simulink model "test_YAN_fusion"  (R2020b)
settings: Solver=ode1  StartTime=t0  StopTime=tf  FixedStep=0.004  RelTol=1e-3  EnableMultiTasking=on
values from neighbouring files (symbols this model uses):
  IMU = IN_SENSOR.IMU1    [run_simulation.m]
undefined symbols (not defined in the file or in its folder): accel_x, accel_y, accel_z, airspeed, airspeed1, airspeed2, airspeed3, airspeed_calibrate, airspeed_indicate, airspeed_true, alt_baro, baro1, baro2, BESTPOS, delta_height, delta_lat, delta_lon, dynamic_pressure, EAS2TAS_Algo, flag, Flag, glv, gyro_x, gyro_y, gyro_z, hAcc, headAcc, height, IMU1, IMU1_Control, IMU2, IMU3, IMU4, laserDown1, laserDown2, Lat, Lon, mag1, mag2, mag_x, mag_y, mag_z, nChange, numSv, pDop, radar1, radarLongDown1, radarLongForward1, range, Range, sAcc, SNR, static_pressure, status, strength, temperature, time, ublox1, um482, vAcc ... (+3)
(part 1 of 3)
settings Model: PauseTimes=[10 20]  Creator=sl  LastModifiedBy=sl
settings SolverCC: AutoInsertRateTranBlk=on
settings OptimizationCC: DefaultParameterBehavior=Inlined  EnhancedBackFolding=on  PassReuseOutputArgsAs=Individual arguments  ZeroExternalMemoryAtStartup=off  ZeroInternalMemoryAtStartup=off  MaxStackSize=64  OptimizeBlockOrder=speed  DifferentSizesBufferReuse=on  OptimizationCustomize=off  EfficientTunableParamExpr=on
settings DebuggingCC: MultiTaskCondExecSysMsg=none  ParameterTunabilityLossMsg=error  UnconnectedInputMsg=none  UnconnectedOutputMsg=none  UnconnectedLineMsg=none
settings HardwareCC: ProdBitPerPointer=32  ProdBitPerSizeT=32  ProdBitPerPtrDiffT=32  ProdLargestAtomicInteger=Long  ProdLargestAtomicFloat=Double  ProdWordSize=32  ProdHWDeviceType=ARM Compatible->ARM Cortex
settings SFSimCC: MATLABDynamicMemAlloc=off
settings RTWCC: Description=Embedded Coder  SystemTargetFile=ert.tlc  TemplateMakefile=ert_default_tmf  GenerateReport=on  IncludeHyperlinkInReport=on  LaunchReport=on  GenerateTraceInfo=on  GenerateTraceReport=on  GenerateTraceReportSl=on  GenerateTraceReportSf=on  GenerateTraceReportEml=on
settings CodeAppCC: ForceParamTrailComments=on  IgnoreCustomStorageClasses=off  OperatorAnnotations=on  SimulinkDataObjDesc=on  SFDataObjDesc=on  InsertBlockDesc=on
settings ERTTargetCC: InlinedParameterPlacement=NonHierarchical  ERTCustomFileTemplate=example_file_process.tlc

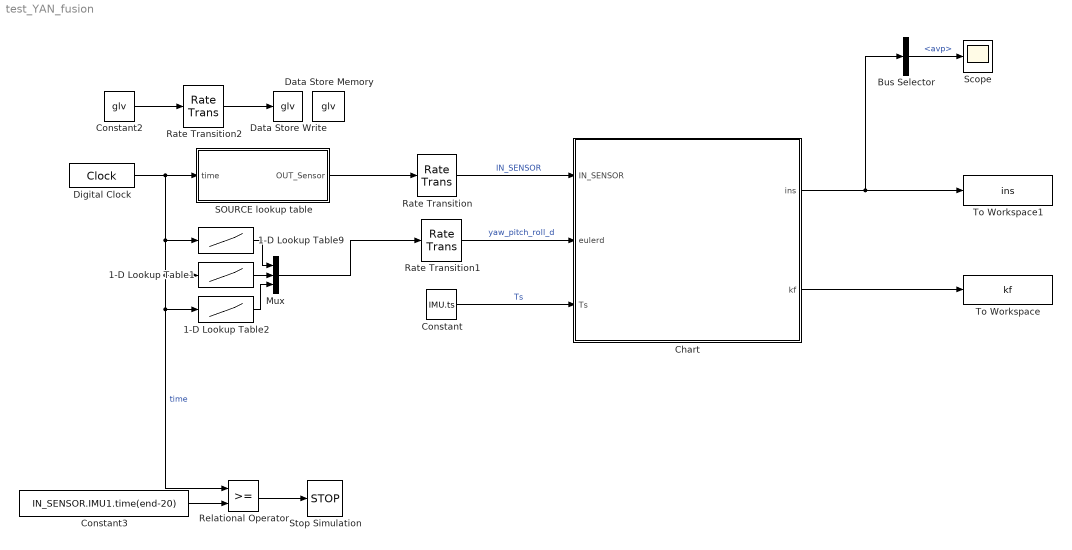
== system test_YAN_fusion ==
  1-D Lookup Table1 : Lookup_n-D  NumberOfTableDimensions=1  BreakpointsForDimension1=FlightLog_Original.Filter.time_cal(1:end-20)  Table=FlightLog_Original.Filter.algo_NAV_pitchd(1:end-20)  InterpMethod=Flat  ExtrapMethod=Clip  InternalRulePriority=Speed  RndMeth=Simplest  InputSameDT=on
  1-D Lookup Table2 : Lookup_n-D  NumberOfTableDimensions=1  BreakpointsForDimension1=FlightLog_Original.Filter.time_cal(1:end-20)  Table=FlightLog_Original.Filter.algo_NAV_rolld(1:end-20)  InterpMethod=Flat  ExtrapMethod=Clip  InternalRulePriority=Speed  RndMeth=Simplest  InputSameDT=on
  1-D Lookup Table9 : Lookup_n-D  NumberOfTableDimensions=1  BreakpointsForDimension1=FlightLog_Original.Filter.time_cal(1:end-20)  Table=FlightLog_Original.Filter.algo_NAV_yawd(1:end-20)  InterpMethod=Flat  ExtrapMethod=Clip  InternalRulePriority=Speed  RndMeth=Simplest  InputSameDT=on
  Bus Selector : BusSelector  OutputSignals=avp
  Chart : Stateflow chart  TreatAsAtomicUnit=on
  Constant : Constant  Value=IMU.ts
  Constant2 : Constant  Value=glv  OutDataTypeStr=Bus: BUS_NAVI_YAN_Glv
  Constant3 : Constant  Value=IN_SENSOR.IMU1.time(end-20)
  Data Store Memory : DataStoreMemory  DataStoreName=glv  ReadBeforeWriteMsg=warning  WriteAfterWriteMsg=warning  WriteAfterReadMsg=warning  ShowAdditionalParam=off  OutDataTypeStr=Bus: BUS_NAVI_YAN_Glv
  Data Store Write : DataStoreWrite  DataStoreName=glv
  Digital Clock : DigitalClock  SampleTime=0.004
  Mux : Mux  Inputs=3
  Rate Transition : RateTransition  OutPortSampleTime=IMU.ts
  Rate Transition1 : RateTransition  OutPortSampleTime=IMU.ts
  Rate Transition2 : RateTransition  OutPortSampleTime=IMU.ts
  Relational Operator : RelationalOperator  OutDataTypeStr=boolean  RndMeth=Simplest
  SOURCE lookup table : Subsystem
  Scope : Scope
  Stop Simulation : Stop
  To Workspace : ToWorkspace  VariableName=kf  SaveFormat=Timeseries  SampleTime=-1
  To Workspace1 : ToWorkspace  VariableName=ins  SaveFormat=Timeseries  SampleTime=-1
  wires:
  Digital Clock/1 -> 1-D Lookup Table1/1, 1-D Lookup Table2/1, Relational Operator/1, 1-D Lookup Table9/1, SOURCE lookup table/1(time)  "time"
  SOURCE lookup table/1(OUT_Sensor) -> Rate Transition/1
  Rate Transition/1 -> Chart/1(IN_SENSOR)  "IN_SENSOR"
  1-D Lookup Table9/1 -> Mux/1
  Constant2/1 -> Rate Transition2/1
  Rate Transition1/1 -> Chart/2(eulerd)  "yaw_pitch_roll_d"
  Rate Transition2/1 -> Data Store Write/1
  Constant/1 -> Chart/3(Ts)  "Ts"
  Chart/2(kf) -> To Workspace/1
  Constant3/1 -> Relational Operator/2
  Relational Operator/1 -> Stop Simulation/1
  Chart/1(ins) -> Bus Selector/1, To Workspace1/1
  Bus Selector/1 -> Scope/1  "<avp>"
  1-D Lookup Table1/1 -> Mux/2
  1-D Lookup Table2/1 -> Mux/3
  Mux/1 -> Rate Transition1/1

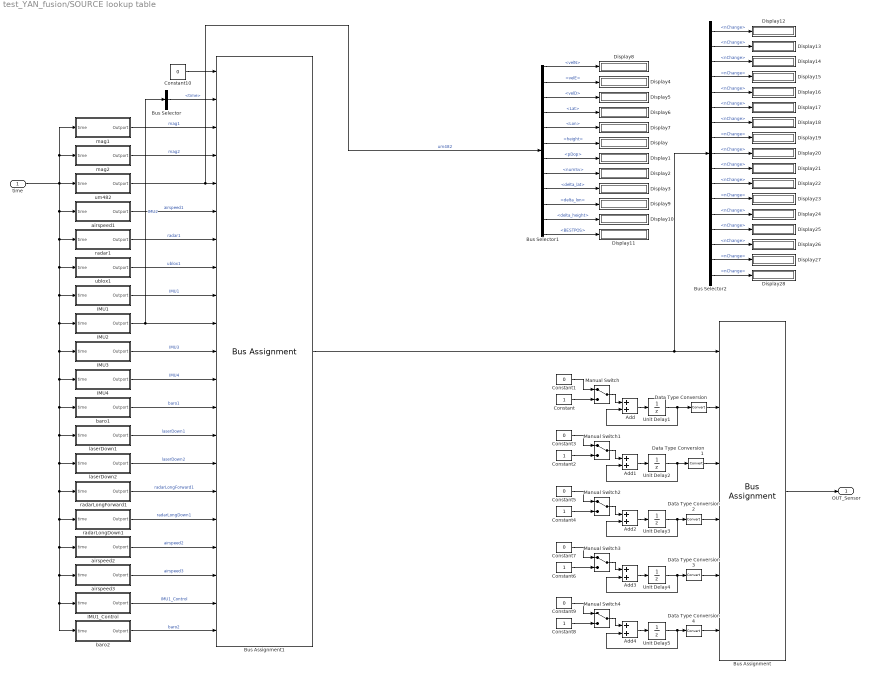
== system test_YAN_fusion/SOURCE lookup table ==
  time : Inport
  Add{,1..4} (5 alike) : Sum
  Bus Assignment : BusAssignment  AssignedSignals=IMU1.nChange,IMU2.nChange,IMU3.nChange,mag1.nChange,mag2.nChange
  Bus Assignment1 : BusAssignment  AssignedSignals=time,mag1,mag2,um482,airspeed1,radar1,ublox1,IMU1,IMU2,IMU3,IMU4,baro1,laserDown1,laserDown2,radarLongForward1,radarLongDown1,airspeed2,airspeed3,IMU1_Control,baro2
  Bus Selector : BusSelector  OutputSignals=time
  Bus Selector1 : BusSelector  OutputSignals=velN,velE,velD,Lat,Lon,height,pDop,numSv,delta_lat,delta_lon,delta_height,BESTPOS
  Bus Selector2 : BusSelector  OutputSignals=mag1.nChange,mag2.nChange,ublox1.nChange,um482.nChange,airspeed1.nChange,airspeed2.nChange,airspeed3.nChange,radar1.nChange,IMU1.nChange,IMU2.nChange,IMU3.nChange,IMU1_Control.nChange,baro1.nChange,laserDown1.nChange,laserDown2.nChange,radarLongForward1.nChange,radarLongDown1.nChange
  Constant{,2,4,6,8} (5 alike) : Constant
  Constant{1,3,5,7,9} (5 alike) : Constant  Value=0
  Constant10 : Constant  Value=0  OutDataTypeStr=Bus: BUS_SENSOR
  Data Type Conversion{,1..4} (5 alike) : DataTypeConversion
  Display{,1..28} (29 alike) : Display
  IMU1 : Subsystem
  IMU1_Control : Subsystem
  IMU2 : Subsystem
  IMU3 : Subsystem
  IMU4 : Subsystem
  Manual Switch{,1..4} (5 alike) : ManualSwitch
  Unit Delay{1..5} (5 alike) : UnitDelay  SampleTime=-1  HasFrameUpgradeWarning=on
  airspeed1 : Subsystem
  airspeed2 : Subsystem
  airspeed3 : Subsystem
  baro1 : Subsystem
  baro2 : Subsystem
  laserDown1 : Subsystem
  laserDown2 : Subsystem
  mag1 : Subsystem
  mag2 : Subsystem
  radar1 : Subsystem
  radarLongDown1 : Subsystem
  radarLongForward1 : Subsystem
  ublox1 : Subsystem
  um482 : Subsystem
  OUT_Sensor : Outport
  wires:
  time/1 -> radarLongForward1/1(time), radarLongDown1/1(time), baro2/1(time), IMU1_Control/1(time), airspeed3/1(time), airspeed2/1(time), laserDown2/1(time), laserDown1/1(time), baro1/1(time), IMU4/1(time), IMU3/1(time), IMU2/1(time), IMU1/1(time), ublox1/1(time), radar1/1(time), airspeed1/1(time), mag2/1(time), mag1/1(time), um482/1(time)
  Bus Selector/1 -> Bus Assignment1/2  "<time>"
  IMU2/1(Outport) -> Bus Assignment1/10, Bus Selector/1  "IMU2"
  ublox1/1(Outport) -> Bus Assignment1/8  "ublox1"
  laserDown2/1(Outport) -> Bus Assignment1/15  "laserDown2"
  IMU3/1(Outport) -> Bus Assignment1/11  "IMU3"
  airspeed2/1(Outport) -> Bus Assignment1/18  "airspeed2"
  um482/1(Outport) -> Bus Assignment1/5, Bus Selector1/1  "um482"
  radarLongDown1/1(Outport) -> Bus Assignment1/17  "radarLongDown1"
  airspeed1/1(Outport) -> Bus Assignment1/6  "airspeed1"
  mag2/1(Outport) -> Bus Assignment1/4  "mag2"
  IMU1/1(Outport) -> Bus Assignment1/9  "IMU1"
  mag1/1(Outport) -> Bus Assignment1/3  "mag1"
  baro1/1(Outport) -> Bus Assignment1/13  "baro1"
  radar1/1(Outport) -> Bus Assignment1/7  "radar1"
  laserDown1/1(Outport) -> Bus Assignment1/14  "laserDown1"
  airspeed3/1(Outport) -> Bus Assignment1/19  "airspeed3"
  IMU1_Control/1(Outport) -> Bus Assignment1/20  "IMU1_Control"
  radarLongForward1/1(Outport) -> Bus Assignment1/16  "radarLongForward1"
  Bus Assignment1/1 -> Bus Selector2/1, Bus Assignment/1
  Bus Selector1/5 -> Display7/1  "<Lon>"
  Bus Selector1/6 -> Display/1  "<height>"
  Bus Selector1/7 -> Display1/1  "<pDop>"
  Bus Selector1/8 -> Display2/1  "<numSv>"
  Bus Selector1/1 -> Display8/1  "<velN>"
  Bus Selector1/2 -> Display4/1  "<velE>"
  Bus Selector1/3 -> Display5/1  "<velD>"
  Bus Selector1/4 -> Display6/1  "<Lat>"
  Bus Selector1/9 -> Display3/1  "<delta_lat>"
  Bus Selector1/10 -> Display9/1  "<delta_lon>"
  Bus Selector1/11 -> Display10/1  "<delta_height>"
  Bus Selector1/12 -> Display11/1  "<BESTPOS>"
  Bus Selector2/1 -> Display12/1  "<nChange>"
  Bus Selector2/2 -> Display13/1  "<nChange>"
  Bus Selector2/3 -> Display14/1  "<nChange>"
  Bus Selector2/4 -> Display15/1  "<nChange>"
  Bus Selector2/5 -> Display16/1  "<nChange>"
  Bus Selector2/6 -> Display17/1  "<nChange>"
  Bus Selector2/7 -> Display18/1  "<nChange>"
  Bus Selector2/8 -> Display19/1  "<nChange>"
  Bus Selector2/9 -> Display20/1  "<nChange>"
  Bus Selector2/10 -> Display21/1  "<nChange>"
  Bus Selector2/11 -> Display22/1  "<nChange>"
  Bus Selector2/12 -> Display23/1  "<nChange>"
  Bus Selector2/13 -> Display24/1  "<nChange>"
  Bus Selector2/14 -> Display25/1  "<nChange>"
  Bus Selector2/15 -> Display26/1  "<nChange>"
  Bus Selector2/16 -> Display27/1  "<nChange>"
  Bus Selector2/17 -> Display28/1  "<nChange>"
  Bus Assignment/1 -> OUT_Sensor/1
  Constant/1 -> Manual Switch/2
  Add/1 -> Unit Delay1/1
  Unit Delay1/1 -> Add/2, Data Type Conversion/1
  Constant1/1 -> Manual Switch/1
  Manual Switch/1 -> Add/1
  Manual Switch1/1 -> Add1/1
  Constant3/1 -> Manual Switch1/1
  Unit Delay2/1 -> Data Type Conversion1/1, Add1/2
  Add1/1 -> Unit Delay2/1
  Constant2/1 -> Manual Switch1/2
  Constant4/1 -> Manual Switch2/2
  Add2/1 -> Unit Delay3/1
  Unit Delay3/1 -> Data Type Conversion2/1, Add2/2
  Constant5/1 -> Manual Switch2/1
  Manual Switch2/1 -> Add2/1
  Data Type Conversion/1 -> Bus Assignment/2
  Data Type Conversion1/1 -> Bus Assignment/3
  Data Type Conversion2/1 -> Bus Assignment/4
  Data Type Conversion3/1 -> Bus Assignment/5
  Manual Switch3/1 -> Add3/1
  Constant7/1 -> Manual Switch3/1
  Unit Delay4/1 -> Add3/2, Data Type Conversion3/1
  Add3/1 -> Unit Delay4/1
  Constant6/1 -> Manual Switch3/2
  Constant8/1 -> Manual Switch4/2
  Add4/1 -> Unit Delay5/1
  Unit Delay5/1 -> Data Type Conversion4/1, Add4/2
  Constant9/1 -> Manual Switch4/1
  Manual Switch4/1 -> Add4/1
  Data Type Conversion4/1 -> Bus Assignment/6
  IMU4/1(Outport) -> Bus Assignment1/12  "IMU4"
  baro2/1(Outport) -> Bus Assignment1/21  "baro2"
  Constant10/1 -> Bus Assignment1/1

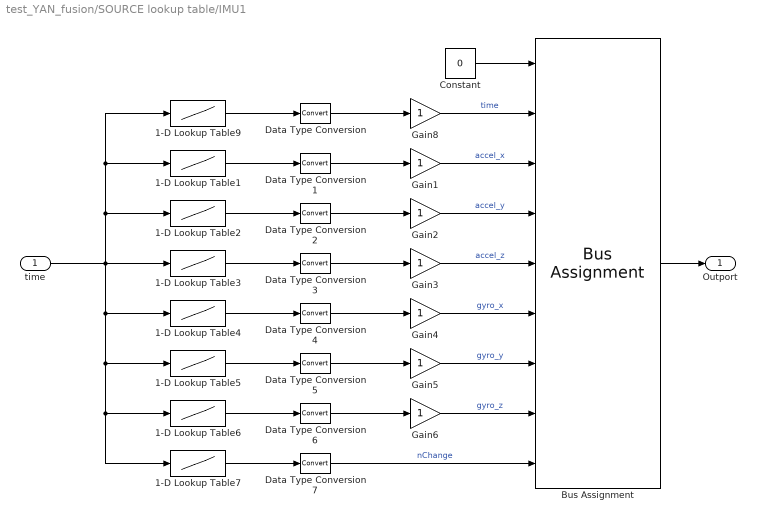
== system test_YAN_fusion/SOURCE lookup table/IMU1 ==
  time : Inport
  1-D Lookup Table1 : Lookup_n-D  NumberOfTableDimensions=1  BreakpointsForDimension1=IN_SENSOR.IMU1.time(1:end-20)  Table=IN_SENSOR.IMU1.accel_x(1:end-20)  InterpMethod=Flat  ExtrapMethod=Clip  InternalRulePriority=Speed  RndMeth=Simplest  InputSameDT=on
  1-D Lookup Table2 : Lookup_n-D  NumberOfTableDimensions=1  BreakpointsForDimension1=IN_SENSOR.IMU1.time(1:end-20)  Table=IN_SENSOR.IMU1.accel_y(1:end-20)  InterpMethod=Flat  ExtrapMethod=Clip  InternalRulePriority=Speed  RndMeth=Simplest  InputSameDT=on
  1-D Lookup Table3 : Lookup_n-D  NumberOfTableDimensions=1  BreakpointsForDimension1=IN_SENSOR.IMU1.time(1:end-20)  Table=IN_SENSOR.IMU1.accel_z(1:end-20)  InterpMethod=Flat  ExtrapMethod=Clip  InternalRulePriority=Speed  RndMeth=Simplest  InputSameDT=on
  1-D Lookup Table4 : Lookup_n-D  NumberOfTableDimensions=1  BreakpointsForDimension1=IN_SENSOR.IMU1.time(1:end-20)  Table=IN_SENSOR.IMU1.gyro_x(1:end-20)  InterpMethod=Flat  ExtrapMethod=Clip  InternalRulePriority=Speed  RndMeth=Simplest  InputSameDT=on
  1-D Lookup Table5 : Lookup_n-D  NumberOfTableDimensions=1  BreakpointsForDimension1=IN_SENSOR.IMU1.time(1:end-20)  Table=IN_SENSOR.IMU1.gyro_y(1:end-20)  InterpMethod=Flat  ExtrapMethod=Clip  InternalRulePriority=Speed  RndMeth=Simplest  InputSameDT=on
  1-D Lookup Table6 : Lookup_n-D  NumberOfTableDimensions=1  BreakpointsForDimension1=IN_SENSOR.IMU1.time(1:end-20)  Table=IN_SENSOR.IMU1.gyro_z(1:end-20)  InterpMethod=Flat  ExtrapMethod=Clip  InternalRulePriority=Speed  RndMeth=Simplest  InputSameDT=on
  1-D Lookup Table7 : Lookup_n-D  NumberOfTableDimensions=1  BreakpointsForDimension1=IN_SENSOR.IMU1.time(1:end-20)  Table=IN_SENSOR.IMU1.nChange(1:end-20)  InterpMethod=Flat  ExtrapMethod=Clip  InternalRulePriority=Speed  RndMeth=Simplest  InputSameDT=on
  1-D Lookup Table9 : Lookup_n-D  NumberOfTableDimensions=1  BreakpointsForDimension1=IN_SENSOR.IMU1.time(1:end-20)  Table=IN_SENSOR.IMU1.time(1:end-20)  InterpMethod=Flat  ExtrapMethod=Clip  InternalRulePriority=Speed  RndMeth=Simplest  InputSameDT=on
  Bus Assignment : BusAssignment  AssignedSignals=time,accel_x,accel_y,accel_z,gyro_x,gyro_y,gyro_z,nChange
  Constant : Constant  Value=0  OutDataTypeStr=Bus: BUS_IMU
  Data Type Conversion{,1..7} (8 alike) : DataTypeConversion
  Gain{1..6,8} (7 alike) : Gain
  Outport : Outport
  wires:
  Gain2/1 -> Bus Assignment/4  "accel_y"
  Gain6/1 -> Bus Assignment/8  "gyro_z"
  Gain3/1 -> Bus Assignment/5  "accel_z"
  Gain4/1 -> Bus Assignment/6  "gyro_x"
  Gain1/1 -> Bus Assignment/3  "accel_x"
  Gain8/1 -> Bus Assignment/2  "time"
  Gain5/1 -> Bus Assignment/7  "gyro_y"
  1-D Lookup Table9/1 -> Data Type Conversion/1
  Data Type Conversion/1 -> Gain8/1
  Data Type Conversion1/1 -> Gain1/1
  1-D Lookup Table1/1 -> Data Type Conversion1/1
  1-D Lookup Table2/1 -> Data Type Conversion2/1
  Data Type Conversion2/1 -> Gain2/1
  Data Type Conversion3/1 -> Gain3/1
  1-D Lookup Table3/1 -> Data Type Conversion3/1
  1-D Lookup Table4/1 -> Data Type Conversion4/1
  Data Type Conversion4/1 -> Gain4/1
  Data Type Conversion5/1 -> Gain5/1
  1-D Lookup Table5/1 -> Data Type Conversion5/1
  1-D Lookup Table6/1 -> Data Type Conversion6/1
  Data Type Conversion6/1 -> Gain6/1
  time/1 -> 1-D Lookup Table7/1, 1-D Lookup Table6/1, 1-D Lookup Table5/1, 1-D Lookup Table4/1, 1-D Lookup Table9/1, 1-D Lookup Table1/1, 1-D Lookup Table2/1, 1-D Lookup Table3/1
  Constant/1 -> Bus Assignment/1
  Bus Assignment/1 -> Outport/1
  1-D Lookup Table7/1 -> Data Type Conversion7/1
  Data Type Conversion7/1 -> Bus Assignment/9  "nChange"

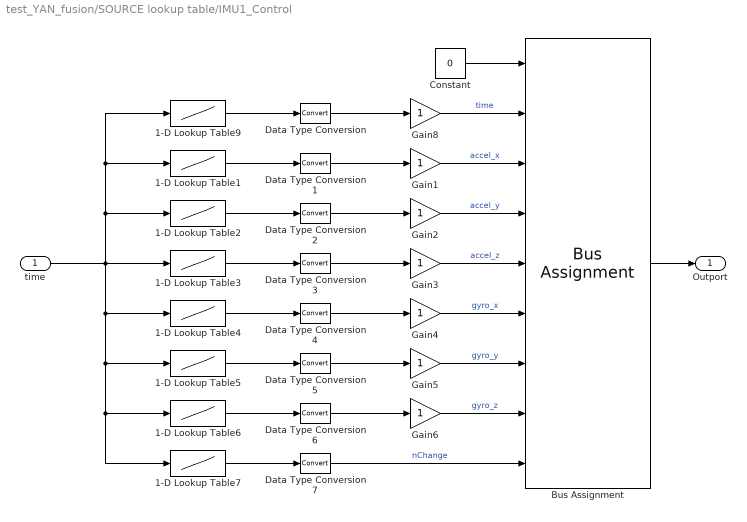
== system test_YAN_fusion/SOURCE lookup table/IMU1_Control ==
  time : Inport
  1-D Lookup Table1 : Lookup_n-D  NumberOfTableDimensions=1  BreakpointsForDimension1=IN_SENSOR.IMU1_Control.time(1:end-20)  Table=IN_SENSOR.IMU1_Control.accel_x(1:end-20)  InterpMethod=Flat  ExtrapMethod=Clip  InternalRulePriority=Speed  RndMeth=Simplest  InputSameDT=on
  1-D Lookup Table2 : Lookup_n-D  NumberOfTableDimensions=1  BreakpointsForDimension1=IN_SENSOR.IMU1_Control.time(1:end-20)  Table=IN_SENSOR.IMU1_Control.accel_y(1:end-20)  InterpMethod=Flat  ExtrapMethod=Clip  InternalRulePriority=Speed  RndMeth=Simplest  InputSameDT=on
  1-D Lookup Table3 : Lookup_n-D  NumberOfTableDimensions=1  BreakpointsForDimension1=IN_SENSOR.IMU1_Control.time(1:end-20)  Table=IN_SENSOR.IMU1_Control.accel_z(1:end-20)  InterpMethod=Flat  ExtrapMethod=Clip  InternalRulePriority=Speed  RndMeth=Simplest  InputSameDT=on
  1-D Lookup Table4 : Lookup_n-D  NumberOfTableDimensions=1  BreakpointsForDimension1=IN_SENSOR.IMU1_Control.time(1:end-20)  Table=IN_SENSOR.IMU1_Control.gyro_x(1:end-20)  InterpMethod=Flat  ExtrapMethod=Clip  InternalRulePriority=Speed  RndMeth=Simplest  InputSameDT=on
  1-D Lookup Table5 : Lookup_n-D  NumberOfTableDimensions=1  BreakpointsForDimension1=IN_SENSOR.IMU1_Control.time(1:end-20)  Table=IN_SENSOR.IMU1_Control.gyro_y(1:end-20)  InterpMethod=Flat  ExtrapMethod=Clip  InternalRulePriority=Speed  RndMeth=Simplest  InputSameDT=on
  1-D Lookup Table6 : Lookup_n-D  NumberOfTableDimensions=1  BreakpointsForDimension1=IN_SENSOR.IMU1_Control.time(1:end-20)  Table=IN_SENSOR.IMU1_Control.gyro_z(1:end-20)  InterpMethod=Flat  ExtrapMethod=Clip  InternalRulePriority=Speed  RndMeth=Simplest  InputSameDT=on
  1-D Lookup Table7 : Lookup_n-D  NumberOfTableDimensions=1  BreakpointsForDimension1=IN_SENSOR.IMU1_Control.time(1:end-20)  Table=IN_SENSOR.IMU1_Control.nChange(1:end-20)  InterpMethod=Flat  ExtrapMethod=Clip  InternalRulePriority=Speed  RndMeth=Simplest  InputSameDT=on
  1-D Lookup Table9 : Lookup_n-D  NumberOfTableDimensions=1  BreakpointsForDimension1=IN_SENSOR.IMU1_Control.time(1:end-20)  Table=IN_SENSOR.IMU1_Control.time(1:end-20)  InterpMethod=Flat  ExtrapMethod=Clip  InternalRulePriority=Speed  RndMeth=Simplest  InputSameDT=on
  Bus Assignment : BusAssignment  AssignedSignals=time,accel_x,accel_y,accel_z,gyro_x,gyro_y,gyro_z,nChange
  Constant : Constant  Value=0  OutDataTypeStr=Bus: BUS_IMU
  Data Type Conversion{,1..7} (8 alike) : DataTypeConversion
  Gain{1..6,8} (7 alike) : Gain
  Outport : Outport
  wires:
  Gain2/1 -> Bus Assignment/4  "accel_y"
  Gain6/1 -> Bus Assignment/8  "gyro_z"
  Gain3/1 -> Bus Assignment/5  "accel_z"
  Gain4/1 -> Bus Assignment/6  "gyro_x"
  Gain1/1 -> Bus Assignment/3  "accel_x"
  Gain8/1 -> Bus Assignment/2  "time"
  Gain5/1 -> Bus Assignment/7  "gyro_y"
  1-D Lookup Table9/1 -> Data Type Conversion/1
  Data Type Conversion/1 -> Gain8/1
  Data Type Conversion1/1 -> Gain1/1
  1-D Lookup Table1/1 -> Data Type Conversion1/1
  1-D Lookup Table2/1 -> Data Type Conversion2/1
  Data Type Conversion2/1 -> Gain2/1
  Data Type Conversion3/1 -> Gain3/1
  1-D Lookup Table3/1 -> Data Type Conversion3/1
  1-D Lookup Table4/1 -> Data Type Conversion4/1
  Data Type Conversion4/1 -> Gain4/1
  Data Type Conversion5/1 -> Gain5/1
  1-D Lookup Table5/1 -> Data Type Conversion5/1
  1-D Lookup Table6/1 -> Data Type Conversion6/1
  Data Type Conversion6/1 -> Gain6/1
  time/1 -> 1-D Lookup Table7/1, 1-D Lookup Table6/1, 1-D Lookup Table5/1, 1-D Lookup Table4/1, 1-D Lookup Table9/1, 1-D Lookup Table1/1, 1-D Lookup Table2/1, 1-D Lookup Table3/1
  Data Type Conversion7/1 -> Bus Assignment/9  "nChange"
  Constant/1 -> Bus Assignment/1
  1-D Lookup Table7/1 -> Data Type Conversion7/1
  Bus Assignment/1 -> Outport/1

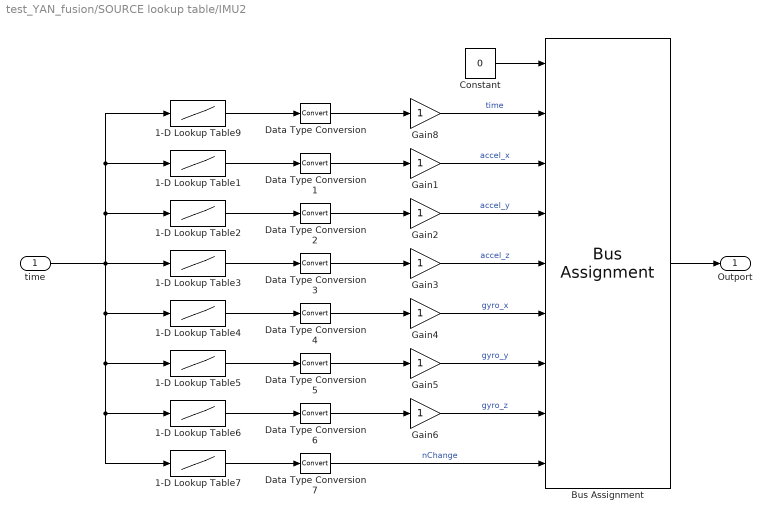
== system test_YAN_fusion/SOURCE lookup table/IMU2 ==
  time : Inport
  1-D Lookup Table1 : Lookup_n-D  NumberOfTableDimensions=1  BreakpointsForDimension1=IN_SENSOR.IMU2.time(1:end-20)  Table=IN_SENSOR.IMU2.accel_x(1:end-20)  InterpMethod=Flat  ExtrapMethod=Clip  InternalRulePriority=Speed  RndMeth=Simplest  InputSameDT=on
  1-D Lookup Table2 : Lookup_n-D  NumberOfTableDimensions=1  BreakpointsForDimension1=IN_SENSOR.IMU2.time(1:end-20)  Table=IN_SENSOR.IMU2.accel_y(1:end-20)  InterpMethod=Flat  ExtrapMethod=Clip  InternalRulePriority=Speed  RndMeth=Simplest  InputSameDT=on
  1-D Lookup Table3 : Lookup_n-D  NumberOfTableDimensions=1  BreakpointsForDimension1=IN_SENSOR.IMU2.time(1:end-20)  Table=IN_SENSOR.IMU2.accel_z(1:end-20)  InterpMethod=Flat  ExtrapMethod=Clip  InternalRulePriority=Speed  RndMeth=Simplest  InputSameDT=on
  1-D Lookup Table4 : Lookup_n-D  NumberOfTableDimensions=1  BreakpointsForDimension1=IN_SENSOR.IMU2.time(1:end-20)  Table=IN_SENSOR.IMU2.gyro_x(1:end-20)  InterpMethod=Flat  ExtrapMethod=Clip  InternalRulePriority=Speed  RndMeth=Simplest  InputSameDT=on
  1-D Lookup Table5 : Lookup_n-D  NumberOfTableDimensions=1  BreakpointsForDimension1=IN_SENSOR.IMU2.time(1:end-20)  Table=IN_SENSOR.IMU2.gyro_y(1:end-20)  InterpMethod=Flat  ExtrapMethod=Clip  InternalRulePriority=Speed  RndMeth=Simplest  InputSameDT=on
  1-D Lookup Table6 : Lookup_n-D  NumberOfTableDimensions=1  BreakpointsForDimension1=IN_SENSOR.IMU2.time(1:end-20)  Table=IN_SENSOR.IMU2.gyro_z(1:end-20)  InterpMethod=Flat  ExtrapMethod=Clip  InternalRulePriority=Speed  RndMeth=Simplest  InputSameDT=on
  1-D Lookup Table7 : Lookup_n-D  NumberOfTableDimensions=1  BreakpointsForDimension1=IN_SENSOR.IMU2.time(1:end-20)  Table=IN_SENSOR.IMU2.nChange(1:end-20)  InterpMethod=Flat  ExtrapMethod=Clip  InternalRulePriority=Speed  RndMeth=Simplest  InputSameDT=on
  1-D Lookup Table9 : Lookup_n-D  NumberOfTableDimensions=1  BreakpointsForDimension1=IN_SENSOR.IMU2.time(1:end-20)  Table=IN_SENSOR.IMU2.time(1:end-20)  InterpMethod=Flat  ExtrapMethod=Clip  InternalRulePriority=Speed  RndMeth=Simplest  InputSameDT=on
  Bus Assignment : BusAssignment  AssignedSignals=time,accel_x,accel_y,accel_z,gyro_x,gyro_y,gyro_z,nChange
  Constant : Constant  Value=0  OutDataTypeStr=Bus: BUS_IMU
  Data Type Conversion{,1..7} (8 alike) : DataTypeConversion
  Gain{1..6,8} (7 alike) : Gain
  Outport : Outport
  wires:
  Data Type Conversion6/1 -> Gain6/1
  1-D Lookup Table6/1 -> Data Type Conversion6/1
  1-D Lookup Table5/1 -> Data Type Conversion5/1
  Data Type Conversion5/1 -> Gain5/1
  Data Type Conversion4/1 -> Gain4/1
  1-D Lookup Table4/1 -> Data Type Conversion4/1
  1-D Lookup Table3/1 -> Data Type Conversion3/1
  Data Type Conversion3/1 -> Gain3/1
  Data Type Conversion2/1 -> Gain2/1
  1-D Lookup Table2/1 -> Data Type Conversion2/1
  1-D Lookup Table1/1 -> Data Type Conversion1/1
  Data Type Conversion1/1 -> Gain1/1
  Data Type Conversion/1 -> Gain8/1
  1-D Lookup Table9/1 -> Data Type Conversion/1
  Gain5/1 -> Bus Assignment/7  "gyro_y"
  Gain8/1 -> Bus Assignment/2  "time"
  Gain1/1 -> Bus Assignment/3  "accel_x"
  Gain4/1 -> Bus Assignment/6  "gyro_x"
  Gain3/1 -> Bus Assignment/5  "accel_z"
  Gain6/1 -> Bus Assignment/8  "gyro_z"
  Gain2/1 -> Bus Assignment/4  "accel_y"
  time/1 -> 1-D Lookup Table3/1, 1-D Lookup Table2/1, 1-D Lookup Table1/1, 1-D Lookup Table9/1, 1-D Lookup Table4/1, 1-D Lookup Table5/1, 1-D Lookup Table7/1, 1-D Lookup Table6/1
  Data Type Conversion7/1 -> Bus Assignment/9  "nChange"
  Constant/1 -> Bus Assignment/1
  1-D Lookup Table7/1 -> Data Type Conversion7/1
  Bus Assignment/1 -> Outport/1

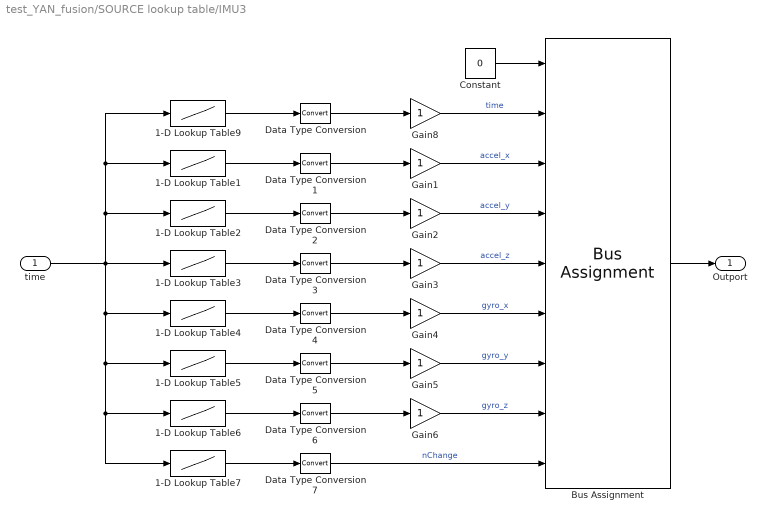
== system test_YAN_fusion/SOURCE lookup table/IMU3 ==
  time : Inport
  1-D Lookup Table1 : Lookup_n-D  NumberOfTableDimensions=1  BreakpointsForDimension1=IN_SENSOR.IMU3.time(1:end-20)  Table=IN_SENSOR.IMU3.accel_x(1:end-20)  InterpMethod=Flat  ExtrapMethod=Clip  InternalRulePriority=Speed  RndMeth=Simplest  InputSameDT=on
  1-D Lookup Table2 : Lookup_n-D  NumberOfTableDimensions=1  BreakpointsForDimension1=IN_SENSOR.IMU3.time(1:end-20)  Table=IN_SENSOR.IMU3.accel_y(1:end-20)  InterpMethod=Flat  ExtrapMethod=Clip  InternalRulePriority=Speed  RndMeth=Simplest  InputSameDT=on
  1-D Lookup Table3 : Lookup_n-D  NumberOfTableDimensions=1  BreakpointsForDimension1=IN_SENSOR.IMU3.time(1:end-20)  Table=IN_SENSOR.IMU3.accel_z(1:end-20)  InterpMethod=Flat  ExtrapMethod=Clip  InternalRulePriority=Speed  RndMeth=Simplest  InputSameDT=on
  1-D Lookup Table4 : Lookup_n-D  NumberOfTableDimensions=1  BreakpointsForDimension1=IN_SENSOR.IMU3.time(1:end-20)  Table=IN_SENSOR.IMU3.gyro_x(1:end-20)  InterpMethod=Flat  ExtrapMethod=Clip  InternalRulePriority=Speed  RndMeth=Simplest  InputSameDT=on
  1-D Lookup Table5 : Lookup_n-D  NumberOfTableDimensions=1  BreakpointsForDimension1=IN_SENSOR.IMU3.time(1:end-20)  Table=IN_SENSOR.IMU3.gyro_y(1:end-20)  InterpMethod=Flat  ExtrapMethod=Clip  InternalRulePriority=Speed  RndMeth=Simplest  InputSameDT=on
  1-D Lookup Table6 : Lookup_n-D  NumberOfTableDimensions=1  BreakpointsForDimension1=IN_SENSOR.IMU3.time(1:end-20)  Table=IN_SENSOR.IMU3.gyro_z(1:end-20)  InterpMethod=Flat  ExtrapMethod=Clip  InternalRulePriority=Speed  RndMeth=Simplest  InputSameDT=on
  1-D Lookup Table7 : Lookup_n-D  NumberOfTableDimensions=1  BreakpointsForDimension1=IN_SENSOR.IMU3.time(1:end-20)  Table=IN_SENSOR.IMU3.nChange(1:end-20)  InterpMethod=Flat  ExtrapMethod=Clip  InternalRulePriority=Speed  RndMeth=Simplest  InputSameDT=on
  1-D Lookup Table9 : Lookup_n-D  NumberOfTableDimensions=1  BreakpointsForDimension1=IN_SENSOR.IMU3.time(1:end-20)  Table=IN_SENSOR.IMU3.time(1:end-20)  InterpMethod=Flat  ExtrapMethod=Clip  InternalRulePriority=Speed  RndMeth=Simplest  InputSameDT=on
  Bus Assignment : BusAssignment  AssignedSignals=time,accel_x,accel_y,accel_z,gyro_x,gyro_y,gyro_z,nChange
  Constant : Constant  Value=0  OutDataTypeStr=Bus: BUS_IMU
  Data Type Conversion{,1..7} (8 alike) : DataTypeConversion
  Gain{1..6,8} (7 alike) : Gain
  Outport : Outport
  wires:
  Gain2/1 -> Bus Assignment/4  "accel_y"
  Gain6/1 -> Bus Assignment/8  "gyro_z"
  Gain3/1 -> Bus Assignment/5  "accel_z"
  Gain4/1 -> Bus Assignment/6  "gyro_x"
  Gain1/1 -> Bus Assignment/3  "accel_x"
  Gain8/1 -> Bus Assignment/2  "time"
  Gain5/1 -> Bus Assignment/7  "gyro_y"
  1-D Lookup Table9/1 -> Data Type Conversion/1
  Data Type Conversion/1 -> Gain8/1
  Data Type Conversion1/1 -> Gain1/1
  1-D Lookup Table1/1 -> Data Type Conversion1/1
  1-D Lookup Table2/1 -> Data Type Conversion2/1
  Data Type Conversion2/1 -> Gain2/1
  Data Type Conversion3/1 -> Gain3/1
  1-D Lookup Table3/1 -> Data Type Conversion3/1
  1-D Lookup Table4/1 -> Data Type Conversion4/1
  Data Type Conversion4/1 -> Gain4/1
  Data Type Conversion5/1 -> Gain5/1
  1-D Lookup Table5/1 -> Data Type Conversion5/1
  1-D Lookup Table6/1 -> Data Type Conversion6/1
  Data Type Conversion6/1 -> Gain6/1
  time/1 -> 1-D Lookup Table7/1, 1-D Lookup Table6/1, 1-D Lookup Table5/1, 1-D Lookup Table4/1, 1-D Lookup Table9/1, 1-D Lookup Table1/1, 1-D Lookup Table2/1, 1-D Lookup Table3/1
  Data Type Conversion7/1 -> Bus Assignment/9  "nChange"
  Constant/1 -> Bus Assignment/1
  1-D Lookup Table7/1 -> Data Type Conversion7/1
  Bus Assignment/1 -> Outport/1

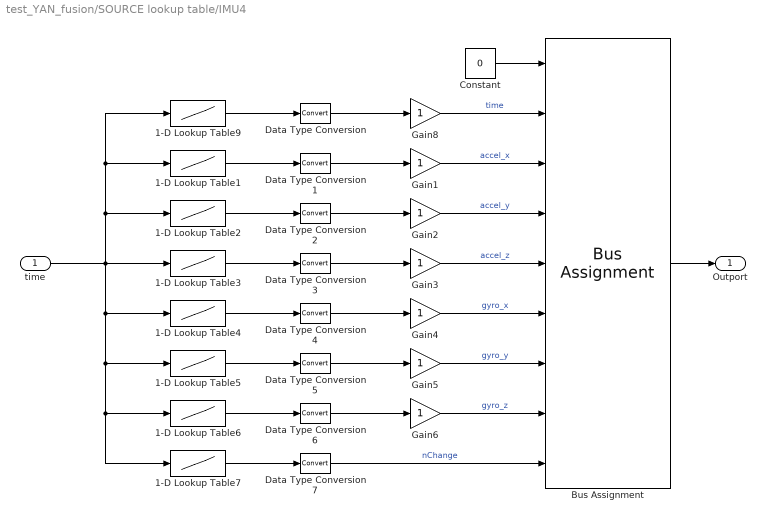
== system test_YAN_fusion/SOURCE lookup table/IMU4 ==
  time : Inport
  1-D Lookup Table1 : Lookup_n-D  NumberOfTableDimensions=1  BreakpointsForDimension1=IN_SENSOR.IMU4.time(1:end-20)  Table=IN_SENSOR.IMU4.accel_x(1:end-20)  InterpMethod=Flat  ExtrapMethod=Clip  InternalRulePriority=Speed  RndMeth=Simplest  InputSameDT=on
  1-D Lookup Table2 : Lookup_n-D  NumberOfTableDimensions=1  BreakpointsForDimension1=IN_SENSOR.IMU4.time(1:end-20)  Table=IN_SENSOR.IMU4.accel_y(1:end-20)  InterpMethod=Flat  ExtrapMethod=Clip  InternalRulePriority=Speed  RndMeth=Simplest  InputSameDT=on
  1-D Lookup Table3 : Lookup_n-D  NumberOfTableDimensions=1  BreakpointsForDimension1=IN_SENSOR.IMU4.time(1:end-20)  Table=IN_SENSOR.IMU4.accel_z(1:end-20)  InterpMethod=Flat  ExtrapMethod=Clip  InternalRulePriority=Speed  RndMeth=Simplest  InputSameDT=on
  1-D Lookup Table4 : Lookup_n-D  NumberOfTableDimensions=1  BreakpointsForDimension1=IN_SENSOR.IMU4.time(1:end-20)  Table=IN_SENSOR.IMU4.gyro_x(1:end-20)  InterpMethod=Flat  ExtrapMethod=Clip  InternalRulePriority=Speed  RndMeth=Simplest  InputSameDT=on
  1-D Lookup Table5 : Lookup_n-D  NumberOfTableDimensions=1  BreakpointsForDimension1=IN_SENSOR.IMU4.time(1:end-20)  Table=IN_SENSOR.IMU4.gyro_y(1:end-20)  InterpMethod=Flat  ExtrapMethod=Clip  InternalRulePriority=Speed  RndMeth=Simplest  InputSameDT=on
  1-D Lookup Table6 : Lookup_n-D  NumberOfTableDimensions=1  BreakpointsForDimension1=IN_SENSOR.IMU4.time(1:end-20)  Table=IN_SENSOR.IMU4.gyro_z(1:end-20)  InterpMethod=Flat  ExtrapMethod=Clip  InternalRulePriority=Speed  RndMeth=Simplest  InputSameDT=on
  1-D Lookup Table7 : Lookup_n-D  NumberOfTableDimensions=1  BreakpointsForDimension1=IN_SENSOR.IMU4.time(1:end-20)  Table=IN_SENSOR.IMU4.nChange(1:end-20)  InterpMethod=Flat  ExtrapMethod=Clip  InternalRulePriority=Speed  RndMeth=Simplest  InputSameDT=on
  1-D Lookup Table9 : Lookup_n-D  NumberOfTableDimensions=1  BreakpointsForDimension1=IN_SENSOR.IMU4.time(1:end-20)  Table=IN_SENSOR.IMU4.time(1:end-20)  InterpMethod=Flat  ExtrapMethod=Clip  InternalRulePriority=Speed  RndMeth=Simplest  InputSameDT=on
  Bus Assignment : BusAssignment  AssignedSignals=time,accel_x,accel_y,accel_z,gyro_x,gyro_y,gyro_z,nChange
  Constant : Constant  Value=0  OutDataTypeStr=Bus: BUS_IMU
  Data Type Conversion{,1..7} (8 alike) : DataTypeConversion
  Gain{1..6,8} (7 alike) : Gain
  Outport : Outport
  wires:
  Bus Assignment/1 -> Outport/1
  1-D Lookup Table7/1 -> Data Type Conversion7/1
  Constant/1 -> Bus Assignment/1
  Data Type Conversion7/1 -> Bus Assignment/9  "nChange"
  time/1 -> 1-D Lookup Table3/1, 1-D Lookup Table2/1, 1-D Lookup Table1/1, 1-D Lookup Table9/1, 1-D Lookup Table4/1, 1-D Lookup Table5/1, 1-D Lookup Table6/1, 1-D Lookup Table7/1
  Data Type Conversion6/1 -> Gain6/1
  1-D Lookup Table6/1 -> Data Type Conversion6/1
  1-D Lookup Table5/1 -> Data Type Conversion5/1
  Data Type Conversion5/1 -> Gain5/1
  Data Type Conversion4/1 -> Gain4/1
  1-D Lookup Table4/1 -> Data Type Conversion4/1
  1-D Lookup Table3/1 -> Data Type Conversion3/1
  Data Type Conversion3/1 -> Gain3/1
  Data Type Conversion2/1 -> Gain2/1
  1-D Lookup Table2/1 -> Data Type Conversion2/1
  1-D Lookup Table1/1 -> Data Type Conversion1/1
  Data Type Conversion1/1 -> Gain1/1
  Data Type Conversion/1 -> Gain8/1
  1-D Lookup Table9/1 -> Data Type Conversion/1
  Gain5/1 -> Bus Assignment/7  "gyro_y"
  Gain8/1 -> Bus Assignment/2  "time"
  Gain1/1 -> Bus Assignment/3  "accel_x"
  Gain4/1 -> Bus Assignment/6  "gyro_x"
  Gain3/1 -> Bus Assignment/5  "accel_z"
  Gain6/1 -> Bus Assignment/8  "gyro_z"
  Gain2/1 -> Bus Assignment/4  "accel_y"

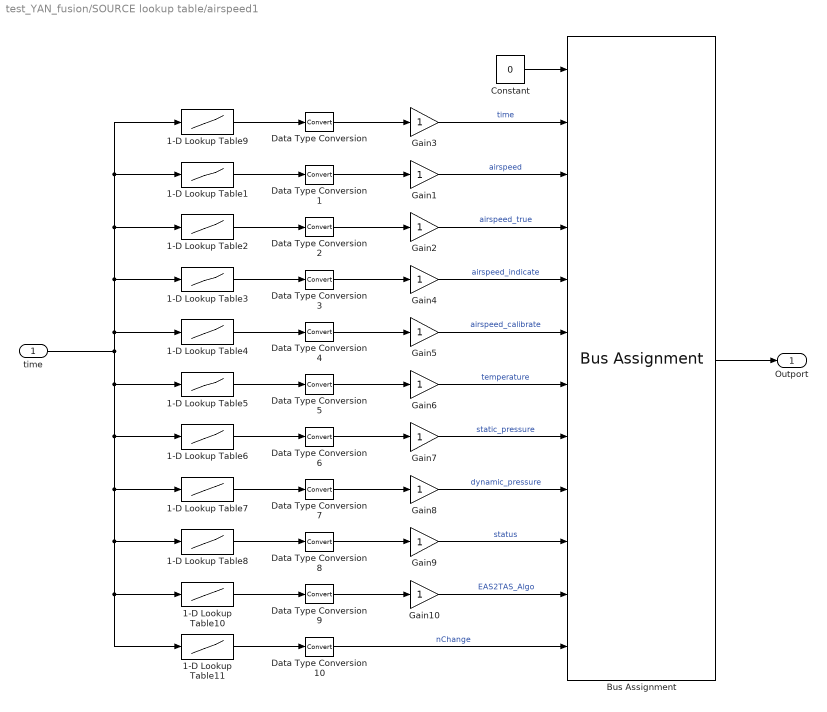
== system test_YAN_fusion/SOURCE lookup table/airspeed1 ==
  time : Inport
  1-D Lookup Table1 : Lookup_n-D  NumberOfTableDimensions=1  BreakpointsForDimension1=IN_SENSOR.airspeed1.time(1:end-20)  Table=IN_SENSOR.airspeed1.airspeed(1:end-20)  InterpMethod=Flat  ExtrapMethod=Clip  InternalRulePriority=Speed  RndMeth=Simplest  InputSameDT=on
  1-D Lookup Table10 : Lookup_n-D  NumberOfTableDimensions=1  BreakpointsForDimension1=IN_SENSOR.airspeed1.time(1:end-20)  Table=IN_SENSOR.airspeed1.EAS2TAS_Algo(1:end-20)  InterpMethod=Flat  ExtrapMethod=Clip  InternalRulePriority=Speed  RndMeth=Simplest  InputSameDT=on
  1-D Lookup Table11 : Lookup_n-D  NumberOfTableDimensions=1  BreakpointsForDimension1=IN_SENSOR.airspeed1.time(1:end-20)  Table=IN_SENSOR.airspeed1.nChange(1:end-20)  InterpMethod=Flat  ExtrapMethod=Clip  InternalRulePriority=Speed  RndMeth=Simplest  InputSameDT=on
  1-D Lookup Table2 : Lookup_n-D  NumberOfTableDimensions=1  BreakpointsForDimension1=IN_SENSOR.airspeed1.time(1:end-20)  Table=IN_SENSOR.airspeed1.airspeed_true(1:end-20)  InterpMethod=Flat  ExtrapMethod=Clip  InternalRulePriority=Speed  RndMeth=Simplest  InputSameDT=on
  1-D Lookup Table3 : Lookup_n-D  NumberOfTableDimensions=1  BreakpointsForDimension1=IN_SENSOR.airspeed1.time(1:end-20)  Table=IN_SENSOR.airspeed1.airspeed_indicate(1:end-20)  InterpMethod=Flat  ExtrapMethod=Clip  InternalRulePriority=Speed  RndMeth=Simplest  InputSameDT=on
  1-D Lookup Table4 : Lookup_n-D  NumberOfTableDimensions=1  BreakpointsForDimension1=IN_SENSOR.airspeed1.time(1:end-20)  Table=IN_SENSOR.airspeed1.airspeed_calibrate(1:end-20)  InterpMethod=Flat  ExtrapMethod=Clip  InternalRulePriority=Speed  RndMeth=Simplest  InputSameDT=on
  1-D Lookup Table5 : Lookup_n-D  NumberOfTableDimensions=1  BreakpointsForDimension1=IN_SENSOR.airspeed1.time(1:end-20)  Table=IN_SENSOR.airspeed1.temperature(1:end-20)  InterpMethod=Flat  ExtrapMethod=Clip  InternalRulePriority=Speed  RndMeth=Simplest  InputSameDT=on
  1-D Lookup Table6 : Lookup_n-D  NumberOfTableDimensions=1  BreakpointsForDimension1=IN_SENSOR.airspeed1.time(1:end-20)  Table=IN_SENSOR.airspeed1.static_pressure(1:end-20)  InterpMethod=Flat  ExtrapMethod=Clip  InternalRulePriority=Speed  RndMeth=Simplest  InputSameDT=on
  1-D Lookup Table7 : Lookup_n-D  NumberOfTableDimensions=1  BreakpointsForDimension1=IN_SENSOR.airspeed1.time(1:end-20)  Table=IN_SENSOR.airspeed1.dynamic_pressure(1:end-20)  InterpMethod=Flat  ExtrapMethod=Clip  InternalRulePriority=Speed  RndMeth=Simplest  InputSameDT=on
  1-D Lookup Table8 : Lookup_n-D  NumberOfTableDimensions=1  BreakpointsForDimension1=IN_SENSOR.airspeed1.time(1:end-20)  Table=IN_SENSOR.airspeed1.status(1:end-20)  InterpMethod=Flat  ExtrapMethod=Clip  InternalRulePriority=Speed  RndMeth=Simplest  InputSameDT=on
  1-D Lookup Table9 : Lookup_n-D  NumberOfTableDimensions=1  BreakpointsForDimension1=IN_SENSOR.airspeed1.time(1:end-20)  Table=IN_SENSOR.airspeed1.time(1:end-20)  InterpMethod=Flat  ExtrapMethod=Clip  InternalRulePriority=Speed  RndMeth=Simplest  InputSameDT=on
  Bus Assignment : BusAssignment  AssignedSignals=time,airspeed,airspeed_true,airspeed_indicate,airspeed_calibrate,temperature,static_pressure,dynamic_pressure,status,EAS2TAS_Algo,nChange
  Constant : Constant  Value=0  OutDataTypeStr=Bus: BUS_AIRSPEED
  Data Type Conversion{,1..10} (11 alike) : DataTypeConversion
  Gain{1..10} (10 alike) : Gain
  Outport : Outport
  wires:
  Gain1/1 -> Bus Assignment/3  "airspeed"
  Gain3/1 -> Bus Assignment/2  "time"
  Gain2/1 -> Bus Assignment/4  "airspeed_true"
  Gain4/1 -> Bus Assignment/5  "airspeed_indicate"
  Gain5/1 -> Bus Assignment/6  "airspeed_calibrate"
  Gain6/1 -> Bus Assignment/7  "temperature"
  Gain7/1 -> Bus Assignment/8  "static_pressure"
  Gain8/1 -> Bus Assignment/9  "dynamic_pressure"
  Gain9/1 -> Bus Assignment/10  "status"
  Gain10/1 -> Bus Assignment/11  "EAS2TAS_Algo"
  Data Type Conversion/1 -> Gain3/1
  1-D Lookup Table9/1 -> Data Type Conversion/1
  1-D Lookup Table1/1 -> Data Type Conversion1/1
  Data Type Conversion1/1 -> Gain1/1
  Data Type Conversion2/1 -> Gain2/1
  1-D Lookup Table2/1 -> Data Type Conversion2/1
  1-D Lookup Table3/1 -> Data Type Conversion3/1
  Data Type Conversion3/1 -> Gain4/1
  Data Type Conversion4/1 -> Gain5/1
  1-D Lookup Table4/1 -> Data Type Conversion4/1
  1-D Lookup Table5/1 -> Data Type Conversion5/1
  Data Type Conversion5/1 -> Gain6/1
  Data Type Conversion6/1 -> Gain7/1
  1-D Lookup Table6/1 -> Data Type Conversion6/1
  1-D Lookup Table7/1 -> Data Type Conversion7/1
  Data Type Conversion7/1 -> Gain8/1
  Data Type Conversion8/1 -> Gain9/1
  1-D Lookup Table8/1 -> Data Type Conversion8/1
  1-D Lookup Table10/1 -> Data Type Conversion9/1
  Data Type Conversion9/1 -> Gain10/1
  time/1 -> 1-D Lookup Table11/1, 1-D Lookup Table10/1, 1-D Lookup Table8/1, 1-D Lookup Table7/1, 1-D Lookup Table6/1, 1-D Lookup Table5/1, 1-D Lookup Table3/1, 1-D Lookup Table9/1, 1-D Lookup Table1/1, 1-D Lookup Table2/1, 1-D Lookup Table4/1
  Constant/1 -> Bus Assignment/1
  Bus Assignment/1 -> Outport/1
  1-D Lookup Table11/1 -> Data Type Conversion10/1
  Data Type Conversion10/1 -> Bus Assignment/12  "nChange"

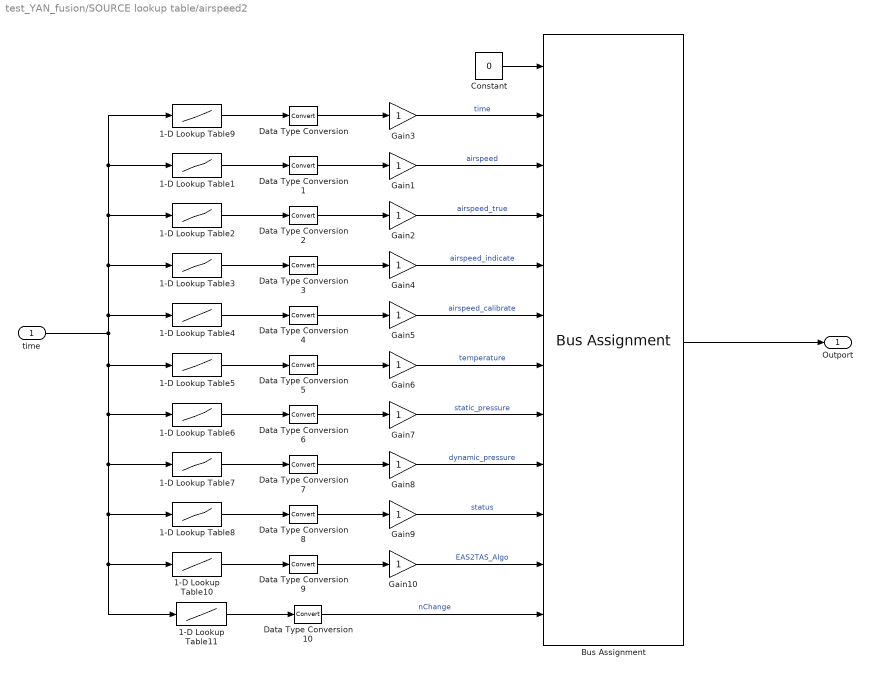
== system test_YAN_fusion/SOURCE lookup table/airspeed2 ==
  time : Inport
  1-D Lookup Table1 : Lookup_n-D  NumberOfTableDimensions=1  BreakpointsForDimension1=IN_SENSOR.airspeed2.time(1:end-20)  Table=IN_SENSOR.airspeed2.airspeed(1:end-20)  InterpMethod=Flat  ExtrapMethod=Clip  InternalRulePriority=Speed  RndMeth=Simplest  InputSameDT=on
  1-D Lookup Table10 : Lookup_n-D  NumberOfTableDimensions=1  BreakpointsForDimension1=IN_SENSOR.airspeed2.time(1:end-20)  Table=IN_SENSOR.airspeed2.EAS2TAS_Algo(1:end-20)  InterpMethod=Flat  ExtrapMethod=Clip  InternalRulePriority=Speed  RndMeth=Simplest  InputSameDT=on
  1-D Lookup Table11 : Lookup_n-D  NumberOfTableDimensions=1  BreakpointsForDimension1=IN_SENSOR.airspeed2.time(1:end-20)  Table=IN_SENSOR.airspeed2.nChange(1:end-20)  InterpMethod=Flat  ExtrapMethod=Clip  InternalRulePriority=Speed  RndMeth=Simplest  InputSameDT=on
  1-D Lookup Table2 : Lookup_n-D  NumberOfTableDimensions=1  BreakpointsForDimension1=IN_SENSOR.airspeed2.time(1:end-20)  Table=IN_SENSOR.airspeed2.airspeed_true(1:end-20)  InterpMethod=Flat  ExtrapMethod=Clip  InternalRulePriority=Speed  RndMeth=Simplest  InputSameDT=on
  1-D Lookup Table3 : Lookup_n-D  NumberOfTableDimensions=1  BreakpointsForDimension1=IN_SENSOR.airspeed2.time(1:end-20)  Table=IN_SENSOR.airspeed2.airspeed_indicate(1:end-20)  InterpMethod=Flat  ExtrapMethod=Clip  InternalRulePriority=Speed  RndMeth=Simplest  InputSameDT=on
  1-D Lookup Table4 : Lookup_n-D  NumberOfTableDimensions=1  BreakpointsForDimension1=IN_SENSOR.airspeed2.time(1:end-20)  Table=IN_SENSOR.airspeed2.airspeed_calibrate(1:end-20)  InterpMethod=Flat  ExtrapMethod=Clip  InternalRulePriority=Speed  RndMeth=Simplest  InputSameDT=on
  1-D Lookup Table5 : Lookup_n-D  NumberOfTableDimensions=1  BreakpointsForDimension1=IN_SENSOR.airspeed2.time(1:end-20)  Table=IN_SENSOR.airspeed2.temperature(1:end-20)  InterpMethod=Flat  ExtrapMethod=Clip  InternalRulePriority=Speed  RndMeth=Simplest  InputSameDT=on
  1-D Lookup Table6 : Lookup_n-D  NumberOfTableDimensions=1  BreakpointsForDimension1=IN_SENSOR.airspeed2.time(1:end-20)  Table=IN_SENSOR.airspeed2.static_pressure(1:end-20)  InterpMethod=Flat  ExtrapMethod=Clip  InternalRulePriority=Speed  RndMeth=Simplest  InputSameDT=on
  1-D Lookup Table7 : Lookup_n-D  NumberOfTableDimensions=1  BreakpointsForDimension1=IN_SENSOR.airspeed2.time(1:end-20)  Table=IN_SENSOR.airspeed2.dynamic_pressure(1:end-20)  InterpMethod=Flat  ExtrapMethod=Clip  InternalRulePriority=Speed  RndMeth=Simplest  InputSameDT=on
  1-D Lookup Table8 : Lookup_n-D  NumberOfTableDimensions=1  BreakpointsForDimension1=IN_SENSOR.airspeed2.time(1:end-20)  Table=IN_SENSOR.airspeed2.status(1:end-20)  InterpMethod=Flat  ExtrapMethod=Clip  InternalRulePriority=Speed  RndMeth=Simplest  InputSameDT=on
  1-D Lookup Table9 : Lookup_n-D  NumberOfTableDimensions=1  BreakpointsForDimension1=IN_SENSOR.airspeed2.time(1:end-20)  Table=IN_SENSOR.airspeed2.time(1:end-20)  InterpMethod=Flat  ExtrapMethod=Clip  InternalRulePriority=Speed  RndMeth=Simplest  InputSameDT=on
  Bus Assignment : BusAssignment  AssignedSignals=time,airspeed,airspeed_true,airspeed_indicate,airspeed_calibrate,temperature,static_pressure,dynamic_pressure,status,EAS2TAS_Algo,nChange
  Constant : Constant  Value=0  OutDataTypeStr=Bus: BUS_AIRSPEED
  Data Type Conversion{,1..10} (11 alike) : DataTypeConversion
  Gain{1..10} (10 alike) : Gain
  Outport : Outport
  wires:
  Gain1/1 -> Bus Assignment/3  "airspeed"
  Gain3/1 -> Bus Assignment/2  "time"
  Gain2/1 -> Bus Assignment/4  "airspeed_true"
  Gain4/1 -> Bus Assignment/5  "airspeed_indicate"
  Gain5/1 -> Bus Assignment/6  "airspeed_calibrate"
  Gain6/1 -> Bus Assignment/7  "temperature"
  Gain7/1 -> Bus Assignment/8  "static_pressure"
  Gain8/1 -> Bus Assignment/9  "dynamic_pressure"
  Gain9/1 -> Bus Assignment/10  "status"
  Gain10/1 -> Bus Assignment/11  "EAS2TAS_Algo"
  Data Type Conversion/1 -> Gain3/1
  1-D Lookup Table9/1 -> Data Type Conversion/1
  1-D Lookup Table1/1 -> Data Type Conversion1/1
  Data Type Conversion1/1 -> Gain1/1
  Data Type Conversion2/1 -> Gain2/1
  1-D Lookup Table2/1 -> Data Type Conversion2/1
  1-D Lookup Table3/1 -> Data Type Conversion3/1
  Data Type Conversion3/1 -> Gain4/1
  Data Type Conversion4/1 -> Gain5/1
  1-D Lookup Table4/1 -> Data Type Conversion4/1
  1-D Lookup Table5/1 -> Data Type Conversion5/1
  Data Type Conversion5/1 -> Gain6/1
  Data Type Conversion6/1 -> Gain7/1
  1-D Lookup Table6/1 -> Data Type Conversion6/1
  1-D Lookup Table7/1 -> Data Type Conversion7/1
  Data Type Conversion7/1 -> Gain8/1
  Data Type Conversion8/1 -> Gain9/1
  1-D Lookup Table8/1 -> Data Type Conversion8/1
  1-D Lookup Table10/1 -> Data Type Conversion9/1
  Data Type Conversion9/1 -> Gain10/1
  Constant/1 -> Bus Assignment/1
  Data Type Conversion10/1 -> Bus Assignment/12  "nChange"
  1-D Lookup Table11/1 -> Data Type Conversion10/1
  time/1 -> 1-D Lookup Table11/1, 1-D Lookup Table10/1, 1-D Lookup Table8/1, 1-D Lookup Table7/1, 1-D Lookup Table6/1, 1-D Lookup Table5/1, 1-D Lookup Table3/1, 1-D Lookup Table9/1, 1-D Lookup Table1/1, 1-D Lookup Table2/1, 1-D Lookup Table4/1
  Bus Assignment/1 -> Outport/1

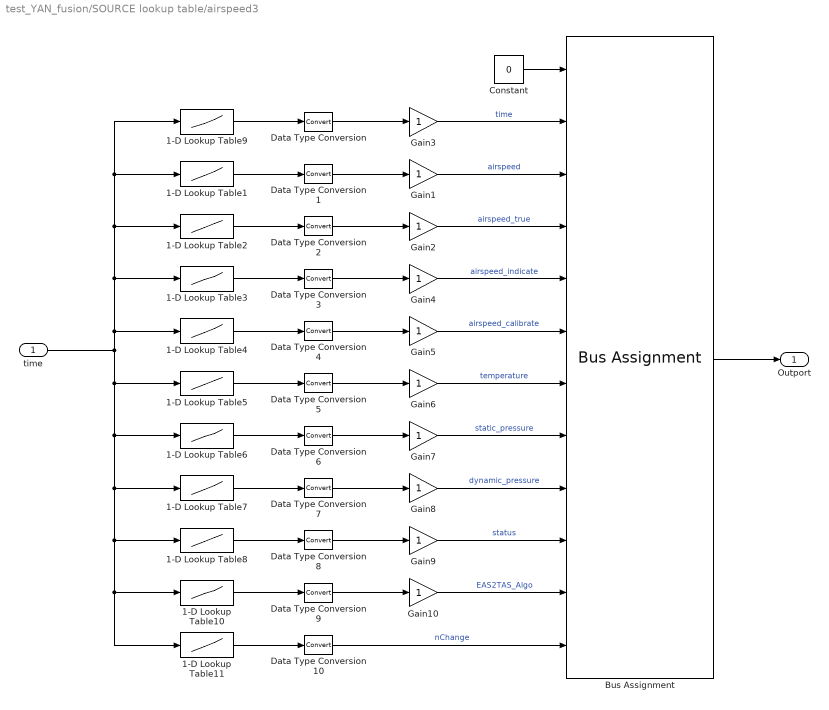
== system test_YAN_fusion/SOURCE lookup table/airspeed3 ==
  time : Inport
  1-D Lookup Table1 : Lookup_n-D  NumberOfTableDimensions=1  BreakpointsForDimension1=IN_SENSOR.airspeed3.time(1:end-20)  Table=IN_SENSOR.airspeed3.airspeed(1:end-20)  InterpMethod=Flat  ExtrapMethod=Clip  InternalRulePriority=Speed  RndMeth=Simplest  InputSameDT=on
  1-D Lookup Table10 : Lookup_n-D  NumberOfTableDimensions=1  BreakpointsForDimension1=IN_SENSOR.airspeed3.time(1:end-20)  Table=IN_SENSOR.airspeed3.EAS2TAS_Algo(1:end-20)  InterpMethod=Flat  ExtrapMethod=Clip  InternalRulePriority=Speed  RndMeth=Simplest  InputSameDT=on
  1-D Lookup Table11 : Lookup_n-D  NumberOfTableDimensions=1  BreakpointsForDimension1=IN_SENSOR.airspeed3.time(1:end-20)  Table=IN_SENSOR.airspeed3.nChange(1:end-20)  InterpMethod=Flat  ExtrapMethod=Clip  InternalRulePriority=Speed  RndMeth=Simplest  InputSameDT=on
  1-D Lookup Table2 : Lookup_n-D  NumberOfTableDimensions=1  BreakpointsForDimension1=IN_SENSOR.airspeed3.time(1:end-20)  Table=IN_SENSOR.airspeed3.airspeed_true(1:end-20)  InterpMethod=Flat  ExtrapMethod=Clip  InternalRulePriority=Speed  RndMeth=Simplest  InputSameDT=on
  1-D Lookup Table3 : Lookup_n-D  NumberOfTableDimensions=1  BreakpointsForDimension1=IN_SENSOR.airspeed3.time(1:end-20)  Table=IN_SENSOR.airspeed3.airspeed_indicate(1:end-20)  InterpMethod=Flat  ExtrapMethod=Clip  InternalRulePriority=Speed  RndMeth=Simplest  InputSameDT=on
  1-D Lookup Table4 : Lookup_n-D  NumberOfTableDimensions=1  BreakpointsForDimension1=IN_SENSOR.airspeed3.time(1:end-20)  Table=IN_SENSOR.airspeed3.airspeed_calibrate(1:end-20)  InterpMethod=Flat  ExtrapMethod=Clip  InternalRulePriority=Speed  RndMeth=Simplest  InputSameDT=on
  1-D Lookup Table5 : Lookup_n-D  NumberOfTableDimensions=1  BreakpointsForDimension1=IN_SENSOR.airspeed3.time(1:end-20)  Table=IN_SENSOR.airspeed3.temperature(1:end-20)  InterpMethod=Flat  ExtrapMethod=Clip  InternalRulePriority=Speed  RndMeth=Simplest  InputSameDT=on
  1-D Lookup Table6 : Lookup_n-D  NumberOfTableDimensions=1  BreakpointsForDimension1=IN_SENSOR.airspeed3.time(1:end-20)  Table=IN_SENSOR.airspeed3.static_pressure(1:end-20)  InterpMethod=Flat  ExtrapMethod=Clip  InternalRulePriority=Speed  RndMeth=Simplest  InputSameDT=on
  1-D Lookup Table7 : Lookup_n-D  NumberOfTableDimensions=1  BreakpointsForDimension1=IN_SENSOR.airspeed3.time(1:end-20)  Table=IN_SENSOR.airspeed3.dynamic_pressure(1:end-20)  InterpMethod=Flat  ExtrapMethod=Clip  InternalRulePriority=Speed  RndMeth=Simplest  InputSameDT=on
  1-D Lookup Table8 : Lookup_n-D  NumberOfTableDimensions=1  BreakpointsForDimension1=IN_SENSOR.airspeed3.time(1:end-20)  Table=IN_SENSOR.airspeed3.status(1:end-20)  InterpMethod=Flat  ExtrapMethod=Clip  InternalRulePriority=Speed  RndMeth=Simplest  InputSameDT=on
  1-D Lookup Table9 : Lookup_n-D  NumberOfTableDimensions=1  BreakpointsForDimension1=IN_SENSOR.airspeed3.time(1:end-20)  Table=IN_SENSOR.airspeed3.time(1:end-20)  InterpMethod=Flat  ExtrapMethod=Clip  InternalRulePriority=Speed  RndMeth=Simplest  InputSameDT=on
  Bus Assignment : BusAssignment  AssignedSignals=time,airspeed,airspeed_true,airspeed_indicate,airspeed_calibrate,temperature,static_pressure,dynamic_pressure,status,EAS2TAS_Algo,nChange
  Constant : Constant  Value=0  OutDataTypeStr=Bus: BUS_AIRSPEED
  Data Type Conversion{,1..10} (11 alike) : DataTypeConversion
  Gain{1..10} (10 alike) : Gain
  Outport : Outport
  wires:
  time/1 -> 1-D Lookup Table4/1, 1-D Lookup Table2/1, 1-D Lookup Table1/1, 1-D Lookup Table9/1, 1-D Lookup Table3/1, 1-D Lookup Table5/1, 1-D Lookup Table6/1, 1-D Lookup Table7/1, 1-D Lookup Table8/1, 1-D Lookup Table11/1, 1-D Lookup Table10/1
  Data Type Conversion9/1 -> Gain10/1
  1-D Lookup Table10/1 -> Data Type Conversion9/1
  1-D Lookup Table8/1 -> Data Type Conversion8/1
  Data Type Conversion8/1 -> Gain9/1
  Data Type Conversion7/1 -> Gain8/1
  1-D Lookup Table7/1 -> Data Type Conversion7/1
  1-D Lookup Table6/1 -> Data Type Conversion6/1
  Data Type Conversion6/1 -> Gain7/1
  Data Type Conversion5/1 -> Gain6/1
  1-D Lookup Table5/1 -> Data Type Conversion5/1
  1-D Lookup Table4/1 -> Data Type Conversion4/1
  Data Type Conversion4/1 -> Gain5/1
  Data Type Conversion3/1 -> Gain4/1
  1-D Lookup Table3/1 -> Data Type Conversion3/1
  1-D Lookup Table2/1 -> Data Type Conversion2/1
  Data Type Conversion2/1 -> Gain2/1
  Data Type Conversion1/1 -> Gain1/1
  1-D Lookup Table1/1 -> Data Type Conversion1/1
  1-D Lookup Table9/1 -> Data Type Conversion/1
  Data Type Conversion/1 -> Gain3/1
  Gain10/1 -> Bus Assignment/11  "EAS2TAS_Algo"
  Gain9/1 -> Bus Assignment/10  "status"
  Gain8/1 -> Bus Assignment/9  "dynamic_pressure"
  Gain7/1 -> Bus Assignment/8  "static_pressure"
  Gain6/1 -> Bus Assignment/7  "temperature"
  Gain5/1 -> Bus Assignment/6  "airspeed_calibrate"
  Gain4/1 -> Bus Assignment/5  "airspeed_indicate"
  Gain2/1 -> Bus Assignment/4  "airspeed_true"
  Gain3/1 -> Bus Assignment/2  "time"
  Gain1/1 -> Bus Assignment/3  "airspeed"
  Data Type Conversion10/1 -> Bus Assignment/12  "nChange"
  1-D Lookup Table11/1 -> Data Type Conversion10/1
  Constant/1 -> Bus Assignment/1
  Bus Assignment/1 -> Outport/1

== system test_YAN_fusion/SOURCE lookup table/baro1 ==
  time : Inport
  1-D Lookup Table1 : Lookup_n-D  NumberOfTableDimensions=1  BreakpointsForDimension1=IN_SENSOR.baro1.time(1:end-20)  Table=IN_SENSOR.baro1.alt_baro(1:end-20)  InterpMethod=Flat  ExtrapMethod=Clip  InternalRulePriority=Speed  RndMeth=Simplest  InputSameDT=on
  1-D Lookup Table2 : Lookup_n-D  NumberOfTableDimensions=1  BreakpointsForDimension1=IN_SENSOR.baro1.time(1:end-20)  Table=IN_SENSOR.baro1.nChange(1:end-20)  InterpMethod=Flat  ExtrapMethod=Clip  InternalRulePriority=Speed  RndMeth=Simplest  InputSameDT=on
  1-D Lookup Table9 : Lookup_n-D  NumberOfTableDimensions=1  BreakpointsForDimension1=IN_SENSOR.baro1.time(1:end-20)  Table=IN_SENSOR.baro1.time(1:end-20)  InterpMethod=Flat  ExtrapMethod=Clip  InternalRulePriority=Speed  RndMeth=Simplest  InputSameDT=on
  Bus Assignment : BusAssignment  AssignedSignals=time,alt_baro,nChange
  Constant : Constant  Value=0  OutDataTypeStr=Bus: BUS_BARO
  Data Type Conversion : DataTypeConversion
  Data Type Conversion1 : DataTypeConversion
  Data Type Conversion2 : DataTypeConversion
  Gain1 : Gain
  Gain8 : Gain
  Outport : Outport
  wires:
  Gain8/1 -> Bus Assignment/2  "time"
  Gain1/1 -> Bus Assignment/3  "alt_baro"
  Data Type Conversion/1 -> Gain8/1
  1-D Lookup Table9/1 -> Data Type Conversion/1
  1-D Lookup Table1/1 -> Data Type Conversion1/1
  Data Type Conversion1/1 -> Gain1/1
  time/1 -> 1-D Lookup Table9/1, 1-D Lookup Table2/1, 1-D Lookup Table1/1
  Constant/1 -> Bus Assignment/1
  1-D Lookup Table2/1 -> Data Type Conversion2/1
  Data Type Conversion2/1 -> Bus Assignment/4  "nChange"
  Bus Assignment/1 -> Outport/1

== system test_YAN_fusion/SOURCE lookup table/baro2 ==
  time : Inport
  1-D Lookup Table1 : Lookup_n-D  NumberOfTableDimensions=1  BreakpointsForDimension1=IN_SENSOR.baro2.time(1:end-20)  Table=IN_SENSOR.baro2.alt_baro(1:end-20)  InterpMethod=Flat  ExtrapMethod=Clip  InternalRulePriority=Speed  RndMeth=Simplest  InputSameDT=on
  1-D Lookup Table2 : Lookup_n-D  NumberOfTableDimensions=1  BreakpointsForDimension1=IN_SENSOR.baro1.time(1:end-20)  Table=IN_SENSOR.baro1.nChange(1:end-20)  InterpMethod=Flat  ExtrapMethod=Clip  InternalRulePriority=Speed  RndMeth=Simplest  InputSameDT=on
  1-D Lookup Table9 : Lookup_n-D  NumberOfTableDimensions=1  BreakpointsForDimension1=IN_SENSOR.baro2.time(1:end-20)  Table=IN_SENSOR.baro2.time(1:end-20)  InterpMethod=Flat  ExtrapMethod=Clip  InternalRulePriority=Speed  RndMeth=Simplest  InputSameDT=on
  Bus Assignment : BusAssignment  AssignedSignals=time,alt_baro,nChange
  Constant : Constant  Value=0  OutDataTypeStr=Bus: BUS_BARO
  Data Type Conversion : DataTypeConversion
  Data Type Conversion1 : DataTypeConversion
  Data Type Conversion2 : DataTypeConversion
  Gain1 : Gain
  Gain8 : Gain
  Outport : Outport
  wires:
  Gain8/1 -> Bus Assignment/2  "time"
  Gain1/1 -> Bus Assignment/3  "alt_baro"
  Data Type Conversion/1 -> Gain8/1
  1-D Lookup Table9/1 -> Data Type Conversion/1
  1-D Lookup Table1/1 -> Data Type Conversion1/1
  Data Type Conversion1/1 -> Gain1/1
  time/1 -> 1-D Lookup Table9/1, 1-D Lookup Table2/1, 1-D Lookup Table1/1
  Constant/1 -> Bus Assignment/1
  1-D Lookup Table2/1 -> Data Type Conversion2/1
  Data Type Conversion2/1 -> Bus Assignment/4  "nChange"
  Bus Assignment/1 -> Outport/1
